simulink model "IDA"  (Simulink 6.0)
settings: Solver=ode45  StartTime=0.0  StopTime=500  RelTol=1e-3
libraries: simulink x6, dspmtrx3 x5
CloseFcn:
  | rtwprivate ssgensfun ModelCloseRequest openloop
settings Model: LastModifiedBy=c chin

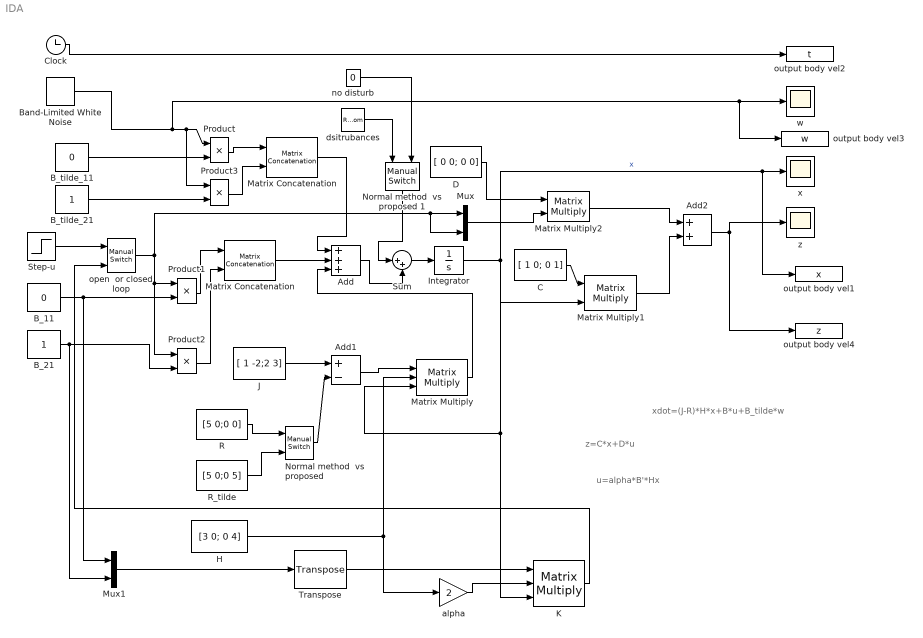
== system IDA ==
  note: xdot=(J-R)*H*x+B*u+B_tilde*w
  note: z=C*x+D*u
  note: u=alpha*B'*Hx
  Add : Sum  Inputs=+++  OutScaling=2^-10
  Add1 : Sum  Inputs=+-  OutScaling=2^-10
  Add2 : Sum  OutScaling=2^-10
  B_11 : Constant  Value=0
  B_21 : Constant
  B_tilde_11 : Constant  Value=0
  B_tilde_21 : Constant
  "Band-Limited White Noise  " : simulink/Sources/Band-Limited White Noise  Cov=[1]  Ts=0.1  seed=[23341]
  C : Constant  Value=[ 1 0; 0 1]
  Clock : Clock
      settings: Decimation=10
  "D " : Constant  Value=[ 0 0; 0 0]
  H : Constant  Value=[3 0; 0 4]
  Integrator : Integrator  InitialCondition=5
  J : Constant  Value=[ 1 -2;2 3]
  K : dspmtrx3/Matrix Multiply  numInputPorts=3  OptimizationLevel=None
  Matrix Concatenation : simulink/Math Operations/Matrix Concatenation  numInports=2  catMethod=Vertical
  "Matrix Concatenation  " : simulink/Math Operations/Matrix Concatenation  numInports=2  catMethod=Vertical
  Matrix Multiply : dspmtrx3/Matrix Multiply  numInputPorts=3  OptimizationLevel=None
  Matrix Multiply1 : dspmtrx3/Matrix Multiply  numInputPorts=2  OptimizationLevel=None
  Matrix Multiply2 : dspmtrx3/Matrix Multiply  numInputPorts=2  OptimizationLevel=None
  Mux : Mux  Inputs=2
  Mux1 : Mux  Inputs=2
  "Normal method  vs proposed " : simulink/Signal Routing/Manual Switch  sw=1  action=0
  Normal method  vs proposed 1 : simulink/Signal Routing/Manual Switch  Orientation=down  sw=1  action=0
  Product{,1..3} (4 alike) : Product  RndMeth=Zero
  R : Constant  Value=[5 0;0 0]
  R_tilde : Constant  Value=[5 0;0 5]
  Step-u : Step  Time=0  After=10  SampleTime=0
  Sum : Sum  Inputs=|++
  Transpose : dspmtrx3/Transpose  Hermitian=off  overflowFlag=on
  alpha : Gain  Gain=2
  dsitrubances : UniformRandomNumber  Minimum=-10  Maximum=10  SampleTime=0
  no disturb : Constant  Value=0
  open  or closed loop : simulink/Signal Routing/Manual Switch  sw=0  action=0
  output body vel1 : ToWorkspace  VariableName=x  SampleTime=1  SaveFormat=Array
  output body vel2 : ToWorkspace  VariableName=t  SampleTime=1  SaveFormat=Array
  output body vel3 : ToWorkspace  VariableName=w  SampleTime=1  SaveFormat=Array
  output body vel4 : ToWorkspace  VariableName=z  SampleTime=1  SaveFormat=Array
  w : Scope
  x : Scope
  z : Scope
      settings: SaveName=ScopeData2
  wires:
  J/1 -> Add1/1
  Add1/1 -> Matrix Multiply/1
  H/1 -> Matrix Multiply/2, alpha/1
  Integrator/1 -> x/1, output body vel1/1, Matrix Multiply1/2, Matrix Multiply/3, K/3  "x"
  R/1 -> "Normal method  vs proposed "/1
  R_tilde/1 -> "Normal method  vs proposed "/2
  "Normal method  vs proposed "/1 -> Add1/2
  Matrix Multiply/1 -> Add/3
  Matrix Concatenation/1 -> Add/1
  "Matrix Concatenation  "/1 -> Add/2
  Product/1 -> Matrix Concatenation/1
  "Band-Limited White Noise  "/1 -> Product/1, Product3/1, w/1, output body vel3/1
  B_11/1 -> Product1/2, Mux1/1
  B_21/1 -> Product2/2, Mux1/2
  Product2/1 -> "Matrix Concatenation  "/2
  Product1/1 -> "Matrix Concatenation  "/1
  B_tilde_11/1 -> Product/2
  Product3/1 -> Matrix Concatenation/2
  B_tilde_21/1 -> Product3/2
  Clock/1 -> output body vel2/1
  Add2/1 -> z/1, output body vel4/1
  Matrix Multiply1/1 -> Add2/2
  C/1 -> Matrix Multiply1/1
  "D "/1 -> Matrix Multiply2/1
  Matrix Multiply2/1 -> Add2/1
  Mux/1 -> Matrix Multiply2/2
  Step-u/1 -> open  or closed loop/1
  open  or closed loop/1 -> Mux/1, Mux/2, Product1/1, Product2/1
  Mux1/1 -> Transpose/1
  Transpose/1 -> K/1
  K/1 -> open  or closed loop/2
  alpha/1 -> K/2
  Add/1 -> Sum/2
  Sum/1 -> Integrator/1
  Normal method  vs proposed 1/1 -> Sum/1
  dsitrubances/1 -> Normal method  vs proposed 1/1
  no disturb/1 -> Normal method  vs proposed 1/2
